simulink model "WaermepumpeGrundlageAnton"  (R2013a)
settings: Solver=ode4  StartTime=0.0  StopTime=1000  FixedStep=1e-1  RelTol=1e-3
StopFcn:
  | ClearSimple
libraries: Thermolib x98, simulink x5
(part 2 of 2)

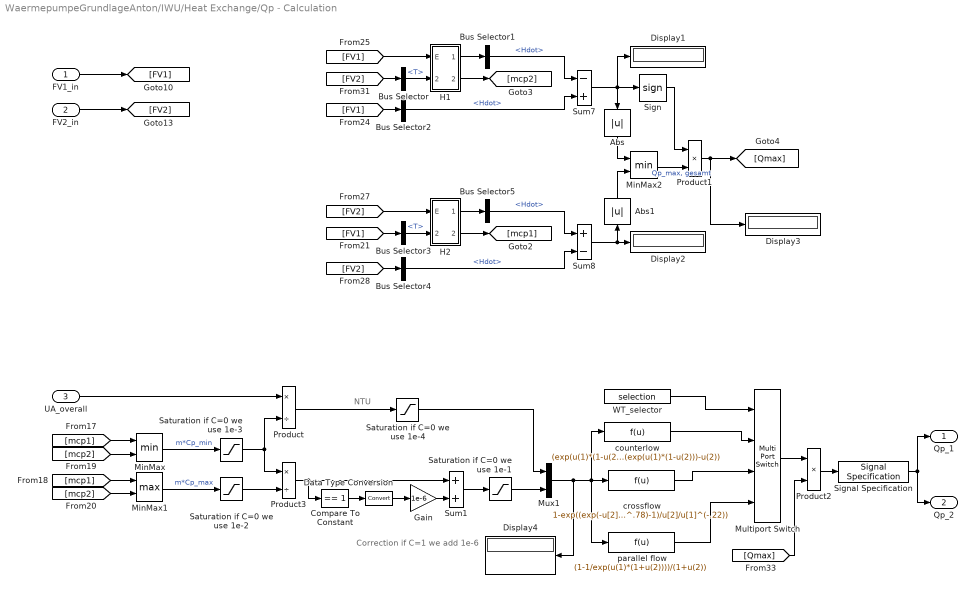
== system WaermepumpeGrundlageAnton/IWU/Heat Exchange/Qp - Calculation ==
  note: Correction if C=1
      | we add 1e-6
  note: NTU
  FV1_in : Inport
  FV2_in : Inport  Port=2
  UA_overall : Inport  Port=3
  Abs : Abs
  Abs1 : Abs
  Bus Selector : BusSelector  OutputSignals=T
  Bus Selector{1..2,4..5} (4 alike) : BusSelector  OutputSignals=Hdot
  Bus Selector3 : BusSelector  OutputSignals=T
  Compare To Constant : simulink/Logic and Bit Operations/Compare To Constant  relop===  const=1  OutDataTypeStr=uint8  ZeroCross=off
  Data Type Conversion : DataTypeConversion
  Display{1..4} (4 alike) : Display
  Gain : Gain  Gain=1e-6
  H1 : Subsystem  TreatAsAtomicUnit=on  mask(H){}
      mask Display: disp('H_g')
  H2 : Subsystem  TreatAsAtomicUnit=on  mask(H){}
      mask Display: disp('H_g')
  MinMax : MinMax  Inputs=2  SaturateOnIntegerOverflow=on  InputSameDT=on
  MinMax1 : MinMax  Function=max  Inputs=2  SaturateOnIntegerOverflow=on  InputSameDT=on
  MinMax2 : MinMax  Inputs=2  SaturateOnIntegerOverflow=on  InputSameDT=on
  Multiport Switch : MultiPortSwitch  SaturateOnIntegerOverflow=on
  Mux1 : Mux  Inputs=2
  Product : Product  Inputs=*/  SaturateOnIntegerOverflow=on  InputSameDT=on  OutDataTypeStr=Inherit: Same as first input
  Product1 : Product  SaturateOnIntegerOverflow=on  InputSameDT=on  OutDataTypeStr=Inherit: Same as first input
  Product2 : Product  SaturateOnIntegerOverflow=on  InputSameDT=on  OutDataTypeStr=Inherit: Same as first input
  Product3 : Product  Inputs=*/  SaturateOnIntegerOverflow=on  InputSameDT=on  OutDataTypeStr=Inherit: Same as first input
  Saturation if C=0 we use 1e-1 : Saturate  UpperLimit=1e19  LowerLimit=1e-19
  Saturation if C=0 we use 1e-2 : Saturate  UpperLimit=1e19  LowerLimit=1e-19
  Saturation if C=0 we use 1e-3 : Saturate  UpperLimit=1e19  LowerLimit=1e-19
  Saturation if C=0 we use 1e-4 : Saturate  UpperLimit=100  LowerLimit=1e-19
  Sign : Signum
  Signal Specification : SignalSpecification  Dimensions=1
  Sum1 : Sum  Inputs=2  SaturateOnIntegerOverflow=on  InputSameDT=on  OutDataTypeStr=Inherit: Same as first input
  Sum7 : Sum  Inputs=-+  SaturateOnIntegerOverflow=on  InputSameDT=on  OutDataTypeStr=Inherit: Same as first input
  Sum8 : Sum  Inputs=+-  SaturateOnIntegerOverflow=on  InputSameDT=on  OutDataTypeStr=Inherit: Same as first input
  WT_selector : Constant  Value=selection
  counterlow : Fcn  Expr=(exp(u(1)*(1-u(2)))-1)/(exp(u(1)*(1-u(2)))-u(2))
  crossflow : Fcn  Expr=1-exp((exp(-u[2]*u[1]^.78)-1)/u[2]/u[1]^(-.22))
  parallel flow : Fcn  Expr=(1-1/exp(u(1)*(1+u(2))))/(1+u(2))
  Qp_1 : Outport
  Qp_2 : Outport  Port=2
  wires:
  Signal Specification/1 -> Qp_2/1, Qp_1/1
  Bus Selector5/1 -> Sum8/1  "<Hdot>"
  Bus Selector4/1 -> Sum8/2  "<Hdot>"
  Bus Selector2/1 -> Sum7/2  "<Hdot>"
  Bus Selector1/1 -> Sum7/1  "<Hdot>"
  Saturation if C=0 we use 1e-1/1 -> Mux1/2
  Saturation if C=0 we use 1e-3/1 -> Product/2, Product3/1
  Saturation if C=0 we use 1e-2/1 -> Product3/2
  Sum1/1 -> Saturation if C=0 we use 1e-1/1
  Gain/1 -> Sum1/2
  Data Type Conversion/1 -> Gain/1
  Compare To Constant/1 -> Data Type Conversion/1
  Product2/1 -> Signal Specification/1
  Mux1/1 -> Display4/1, counterlow/1, parallel flow/1, crossflow/1
  Product3/1 -> Sum1/1, Compare To Constant/1
  MinMax1/1 -> Saturation if C=0 we use 1e-2/1  "m*Cp_max"
  FV1_in/1 -> [FV1]
  FV2_in/1 -> [FV2]
  Product/1 -> Saturation if C=0 we use 1e-4/1
  MinMax/1 -> Saturation if C=0 we use 1e-3/1  "m*Cp_min"
  [mcp1] -> MinMax/1
  [mcp1] -> MinMax1/1
  [mcp2] -> MinMax1/2
  [mcp2] -> MinMax/2
  [Qmax] -> Product2/2
  Multiport Switch/1 -> Product2/1
  counterlow/1 -> Multiport Switch/2
  crossflow/1 -> Multiport Switch/3
  parallel flow/1 -> Multiport Switch/4
  WT_selector/1 -> Multiport Switch/1
  Bus Selector/1 -> H1/2(Temp)  "<T>"
  Bus Selector3/1 -> H2/2(Temp)  "<T>"
  [FV2] -> Bus Selector/1
  [FV2] -> Bus Selector4/1
  [FV2] -> H2/1(E)
  [FV1] -> H1/1(E)
  [FV1] -> Bus Selector2/1
  [FV1] -> Bus Selector3/1
  Sum8/1 -> Abs1/1, Display2/1
  H2/1(FB_out) -> Bus Selector5/1
  Sum7/1 -> Abs/1, Sign/1, Display1/1
  H1/1(FB_out) -> Bus Selector1/1
  MinMax2/1 -> Product1/2  "Qp_max, gesamt"
  Sign/1 -> Product1/1
  Abs/1 -> MinMax2/1
  Abs1/1 -> MinMax2/2
  Product1/1 -> [Qmax], Display3/1
  H2/2(Cp) -> [mcp1]
  H1/2(Cp) -> [mcp2]
  Saturation if C=0 we use 1e-4/1 -> Mux1/1
  UA_overall/1 -> Product/1

== system WaermepumpeGrundlageAnton/IWU/Heat Exchange/first media ==
  Qp : Inport
  FB1_in : Inport  Port=2
  Bus Assignment : BusAssignment  AssignedSignals=Hdot
  Bus Selector : BusSelector  OutputSignals=Hdot
  H-p-State with HeatLoss : Thermolib/Thermodynamic States and Properties/H-p-State with Heat Exchange  k=k_env  A_total=A_env/4  T_env=T_env  relaxation_factor=0.01  conv_limit=TH_THERM_H_P_STATE_T_CONV_LIMIT  hm_conv_limit=TH_THERM_H_P_STATE_HM_CONV_LIMIT  n_iteration=TH_THERM_H_P_STATE_NUM_ITER_MAX  T_initial=T_initial  H_initial=0  ndot_zero_eps=TH_THERM_NDOT_MIN
  Sum7 : Sum  Inputs=2  SaturateOnIntegerOverflow=on  InputSameDT=on  OutDataTypeStr=Inherit: Same as first input
  Terminator4 : Terminator
  FB1_out : Outport
  Q_env : Outport  Port=2
  wires:
  Bus Assignment/1 -> H-p-State with HeatLoss/1
  H-p-State with HeatLoss/2 -> Q_env/1
  H-p-State with HeatLoss/1 -> FB1_out/1
  Bus Selector/1 -> Sum7/2  "<Hdot>"
  Sum7/1 -> Bus Assignment/2
  Qp/1 -> Sum7/1
  FB1_in/1 -> Bus Assignment/1, Bus Selector/1
  H-p-State with HeatLoss/3 -> Terminator4/1

== system WaermepumpeGrundlageAnton/IWU/Heat Exchange/second media ==
  Qp : Inport
  FB2_in : Inport  Port=2
  Bus Assignment : BusAssignment  AssignedSignals=Hdot
  Bus Selector : BusSelector  OutputSignals=Hdot
  H-p-State with HeatLoss1 : Thermolib/Thermodynamic States and Properties/H-p-State with Heat Exchange  k=k_env  A_total=A_env/4  T_env=T_env  relaxation_factor=0.01  conv_limit=TH_THERM_H_P_STATE_T_CONV_LIMIT  hm_conv_limit=TH_THERM_H_P_STATE_HM_CONV_LIMIT  n_iteration=TH_THERM_H_P_STATE_NUM_ITER_MAX  T_initial=T_initial  H_initial=0  ndot_zero_eps=TH_THERM_NDOT_MIN
  Sum1 : Sum  Inputs=2  SaturateOnIntegerOverflow=on  InputSameDT=on  OutDataTypeStr=Inherit: Same as first input
  Terminator4 : Terminator
  FB2_out : Outport
  Q_env : Outport  Port=2
  wires:
  Bus Selector/1 -> Sum1/2  "<Hdot>"
  Bus Assignment/1 -> H-p-State with HeatLoss1/1
  H-p-State with HeatLoss1/2 -> Q_env/1
  FB2_in/1 -> Bus Assignment/1, Bus Selector/1
  Qp/1 -> Sum1/1
  Sum1/1 -> Bus Assignment/2
  H-p-State with HeatLoss1/1 -> FB2_out/1
  H-p-State with HeatLoss1/3 -> Terminator4/1

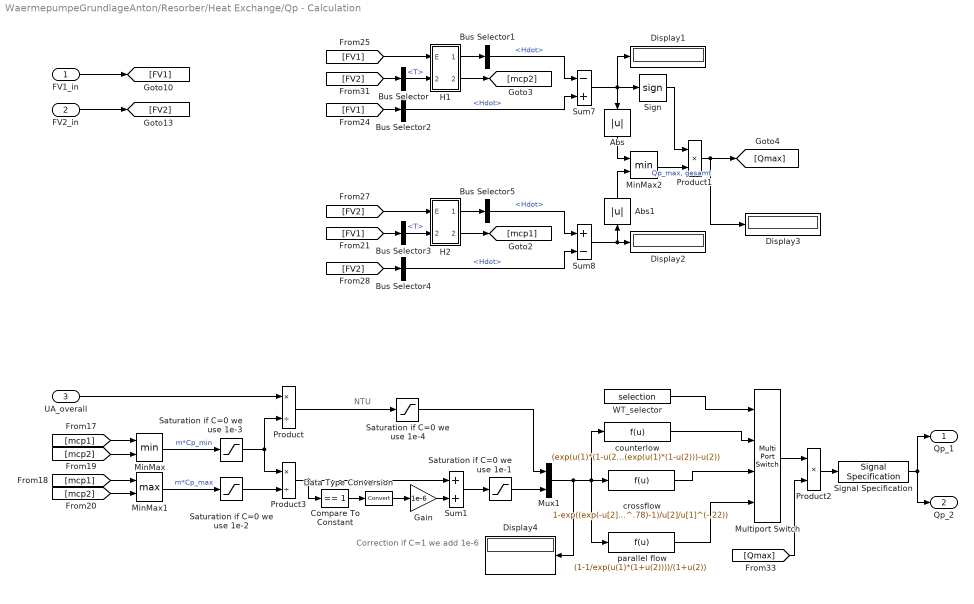
== system WaermepumpeGrundlageAnton/Resorber/Heat Exchange/Qp - Calculation ==
  note: NTU
  note: Correction if C=1
      | we add 1e-6
  FV1_in : Inport
  FV2_in : Inport  Port=2
  UA_overall : Inport  Port=3
  Abs : Abs
  Abs1 : Abs
  Bus Selector : BusSelector  OutputSignals=T
  Bus Selector{1..2,4..5} (4 alike) : BusSelector  OutputSignals=Hdot
  Bus Selector3 : BusSelector  OutputSignals=T
  Compare To Constant : simulink/Logic and Bit Operations/Compare To Constant  relop===  const=1  OutDataTypeStr=uint8  ZeroCross=off
  Data Type Conversion : DataTypeConversion
  Display{1..4} (4 alike) : Display
  Gain : Gain  Gain=1e-6
  H1 : Subsystem  TreatAsAtomicUnit=on  mask(H){}
      mask Display: disp('H_g')
  H2 : Subsystem  TreatAsAtomicUnit=on  mask(H){}
      mask Display: disp('H_g')
  MinMax : MinMax  Inputs=2  SaturateOnIntegerOverflow=on  InputSameDT=on
  MinMax1 : MinMax  Function=max  Inputs=2  SaturateOnIntegerOverflow=on  InputSameDT=on
  MinMax2 : MinMax  Inputs=2  SaturateOnIntegerOverflow=on  InputSameDT=on
  Multiport Switch : MultiPortSwitch  SaturateOnIntegerOverflow=on
  Mux1 : Mux  Inputs=2
  Product : Product  Inputs=*/  SaturateOnIntegerOverflow=on  InputSameDT=on  OutDataTypeStr=Inherit: Same as first input
  Product1 : Product  SaturateOnIntegerOverflow=on  InputSameDT=on  OutDataTypeStr=Inherit: Same as first input
  Product2 : Product  SaturateOnIntegerOverflow=on  InputSameDT=on  OutDataTypeStr=Inherit: Same as first input
  Product3 : Product  Inputs=*/  SaturateOnIntegerOverflow=on  InputSameDT=on  OutDataTypeStr=Inherit: Same as first input
  Saturation if C=0 we use 1e-1 : Saturate  UpperLimit=1e19  LowerLimit=1e-19
  Saturation if C=0 we use 1e-2 : Saturate  UpperLimit=1e19  LowerLimit=1e-19
  Saturation if C=0 we use 1e-3 : Saturate  UpperLimit=1e19  LowerLimit=1e-19
  Saturation if C=0 we use 1e-4 : Saturate  UpperLimit=100  LowerLimit=1e-19
  Sign : Signum
  Signal Specification : SignalSpecification  Dimensions=1
  Sum1 : Sum  Inputs=2  SaturateOnIntegerOverflow=on  InputSameDT=on  OutDataTypeStr=Inherit: Same as first input
  Sum7 : Sum  Inputs=-+  SaturateOnIntegerOverflow=on  InputSameDT=on  OutDataTypeStr=Inherit: Same as first input
  Sum8 : Sum  Inputs=+-  SaturateOnIntegerOverflow=on  InputSameDT=on  OutDataTypeStr=Inherit: Same as first input
  WT_selector : Constant  Value=selection
  counterlow : Fcn  Expr=(exp(u(1)*(1-u(2)))-1)/(exp(u(1)*(1-u(2)))-u(2))
  crossflow : Fcn  Expr=1-exp((exp(-u[2]*u[1]^.78)-1)/u[2]/u[1]^(-.22))
  parallel flow : Fcn  Expr=(1-1/exp(u(1)*(1+u(2))))/(1+u(2))
  Qp_1 : Outport
  Qp_2 : Outport  Port=2
  wires:
  UA_overall/1 -> Product/1
  Saturation if C=0 we use 1e-4/1 -> Mux1/1
  H1/2(Cp) -> [mcp2]
  H2/2(Cp) -> [mcp1]
  Product1/1 -> Display3/1, [Qmax]
  Abs1/1 -> MinMax2/2
  Abs/1 -> MinMax2/1
  Sign/1 -> Product1/1
  MinMax2/1 -> Product1/2  "Qp_max, gesamt"
  H1/1(FB_out) -> Bus Selector1/1
  Sum7/1 -> Display1/1, Sign/1, Abs/1
  H2/1(FB_out) -> Bus Selector5/1
  Sum8/1 -> Display2/1, Abs1/1
  [FV1] -> Bus Selector3/1
  [FV1] -> Bus Selector2/1
  [FV1] -> H1/1(E)
  [FV2] -> H2/1(E)
  [FV2] -> Bus Selector4/1
  [FV2] -> Bus Selector/1
  Bus Selector3/1 -> H2/2(Temp)  "<T>"
  Bus Selector/1 -> H1/2(Temp)  "<T>"
  WT_selector/1 -> Multiport Switch/1
  parallel flow/1 -> Multiport Switch/4
  crossflow/1 -> Multiport Switch/3
  counterlow/1 -> Multiport Switch/2
  Multiport Switch/1 -> Product2/1
  [Qmax] -> Product2/2
  [mcp2] -> MinMax/2
  [mcp2] -> MinMax1/2
  [mcp1] -> MinMax1/1
  [mcp1] -> MinMax/1
  MinMax/1 -> Saturation if C=0 we use 1e-3/1  "m*Cp_min"
  Product/1 -> Saturation if C=0 we use 1e-4/1
  FV2_in/1 -> [FV2]
  FV1_in/1 -> [FV1]
  MinMax1/1 -> Saturation if C=0 we use 1e-2/1  "m*Cp_max"
  Product3/1 -> Compare To Constant/1, Sum1/1
  Mux1/1 -> crossflow/1, parallel flow/1, counterlow/1, Display4/1
  Product2/1 -> Signal Specification/1
  Compare To Constant/1 -> Data Type Conversion/1
  Data Type Conversion/1 -> Gain/1
  Gain/1 -> Sum1/2
  Sum1/1 -> Saturation if C=0 we use 1e-1/1
  Saturation if C=0 we use 1e-2/1 -> Product3/2
  Saturation if C=0 we use 1e-3/1 -> Product3/1, Product/2
  Saturation if C=0 we use 1e-1/1 -> Mux1/2
  Bus Selector1/1 -> Sum7/1  "<Hdot>"
  Bus Selector2/1 -> Sum7/2  "<Hdot>"
  Bus Selector4/1 -> Sum8/2  "<Hdot>"
  Bus Selector5/1 -> Sum8/1  "<Hdot>"
  Signal Specification/1 -> Qp_1/1, Qp_2/1

== system WaermepumpeGrundlageAnton/Resorber/Heat Exchange/first media ==
  Qp : Inport
  FB1_in : Inport  Port=2
  Bus Assignment : BusAssignment  AssignedSignals=Hdot
  Bus Selector : BusSelector  OutputSignals=Hdot
  H-p-State with HeatLoss : Thermolib/Thermodynamic States and Properties/H-p-State with Heat Exchange  k=k_env  A_total=A_env/4  T_env=T_env  relaxation_factor=0.01  conv_limit=TH_THERM_H_P_STATE_T_CONV_LIMIT  hm_conv_limit=TH_THERM_H_P_STATE_HM_CONV_LIMIT  n_iteration=TH_THERM_H_P_STATE_NUM_ITER_MAX  T_initial=T_initial  H_initial=0  ndot_zero_eps=TH_THERM_NDOT_MIN
  Sum7 : Sum  Inputs=2  SaturateOnIntegerOverflow=on  InputSameDT=on  OutDataTypeStr=Inherit: Same as first input
  Terminator4 : Terminator
  FB1_out : Outport
  Q_env : Outport  Port=2
  wires:
  H-p-State with HeatLoss/3 -> Terminator4/1
  FB1_in/1 -> Bus Selector/1, Bus Assignment/1
  Qp/1 -> Sum7/1
  Sum7/1 -> Bus Assignment/2
  Bus Selector/1 -> Sum7/2  "<Hdot>"
  H-p-State with HeatLoss/1 -> FB1_out/1
  H-p-State with HeatLoss/2 -> Q_env/1
  Bus Assignment/1 -> H-p-State with HeatLoss/1

== system WaermepumpeGrundlageAnton/Resorber/Heat Exchange/second media ==
  Qp : Inport
  FB2_in : Inport  Port=2
  Bus Assignment : BusAssignment  AssignedSignals=Hdot
  Bus Selector : BusSelector  OutputSignals=Hdot
  H-p-State with HeatLoss1 : Thermolib/Thermodynamic States and Properties/H-p-State with Heat Exchange  k=k_env  A_total=A_env/4  T_env=T_env  relaxation_factor=0.01  conv_limit=TH_THERM_H_P_STATE_T_CONV_LIMIT  hm_conv_limit=TH_THERM_H_P_STATE_HM_CONV_LIMIT  n_iteration=TH_THERM_H_P_STATE_NUM_ITER_MAX  T_initial=T_initial  H_initial=0  ndot_zero_eps=TH_THERM_NDOT_MIN
  Sum1 : Sum  Inputs=2  SaturateOnIntegerOverflow=on  InputSameDT=on  OutDataTypeStr=Inherit: Same as first input
  Terminator4 : Terminator
  FB2_out : Outport
  Q_env : Outport  Port=2
  wires:
  H-p-State with HeatLoss1/3 -> Terminator4/1
  H-p-State with HeatLoss1/1 -> FB2_out/1
  Sum1/1 -> Bus Assignment/2
  Qp/1 -> Sum1/1
  FB2_in/1 -> Bus Selector/1, Bus Assignment/1
  H-p-State with HeatLoss1/2 -> Q_env/1
  Bus Assignment/1 -> H-p-State with HeatLoss1/1
  Bus Selector/1 -> Sum1/2  "<Hdot>"

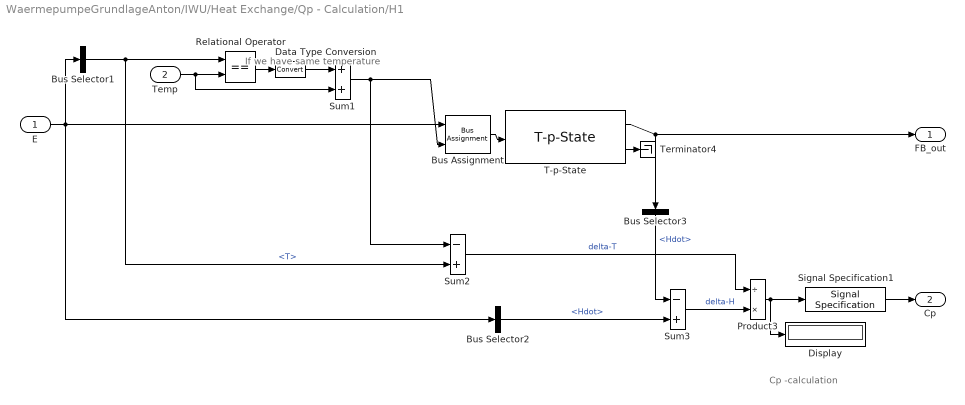
== system WaermepumpeGrundlageAnton/IWU/Heat Exchange/Qp - Calculation/H1 ==
  note: If we have same temperature
  note: Cp -calculation
  E : Inport
  Temp : Inport  Port=2
  Bus Assignment : BusAssignment  AssignedSignals=T
  Bus Selector1 : BusSelector  OutputSignals=T
  Bus Selector2 : BusSelector  OutputSignals=Hdot
  Bus Selector3 : BusSelector  OutputSignals=Hdot
  Data Type Conversion : DataTypeConversion
  Display : Display
  Product3 : Product  Inputs=/*  SaturateOnIntegerOverflow=on  InputSameDT=on  OutDataTypeStr=Inherit: Same as first input
  Relational Operator : RelationalOperator  Operator===  OutDataTypeStr=boolean
  Signal Specification1 : SignalSpecification  Dimensions=1
  Sum1 : Sum  Inputs=2  SaturateOnIntegerOverflow=on  InputSameDT=on  OutDataTypeStr=Inherit: Same as first input
  Sum2 : Sum  Inputs=-+  SaturateOnIntegerOverflow=on  InputSameDT=on  OutDataTypeStr=Inherit: Same as first input
  Sum3 : Sum  Inputs=-+  SaturateOnIntegerOverflow=on  InputSameDT=on  OutDataTypeStr=Inherit: Same as first input
  T-p-State : Thermolib/Thermodynamic States and Properties/T-p-State
  Terminator4 : Terminator
  FB_out : Outport
  Cp : Outport  Port=2
  wires:
  Signal Specification1/1 -> Cp/1
  Bus Selector3/1 -> Sum3/1  "<Hdot>"
  Bus Selector2/1 -> Sum3/2  "<Hdot>"
  Product3/1 -> Signal Specification1/1, Display/1
  Sum2/1 -> Product3/1  "delta-T"
  Sum3/1 -> Product3/2  "delta-H"
  Data Type Conversion/1 -> Sum1/1
  Relational Operator/1 -> Data Type Conversion/1
  Temp/1 -> Sum1/2, Relational Operator/2
  E/1 -> Bus Assignment/1, Bus Selector2/1, Bus Selector1/1
  T-p-State/1 -> Bus Selector3/1, FB_out/1
  Bus Assignment/1 -> T-p-State/1
  Bus Selector1/1 -> Sum2/2, Relational Operator/1  "<T>"
  Sum1/1 -> Sum2/1, Bus Assignment/2
  T-p-State/2 -> Terminator4/1

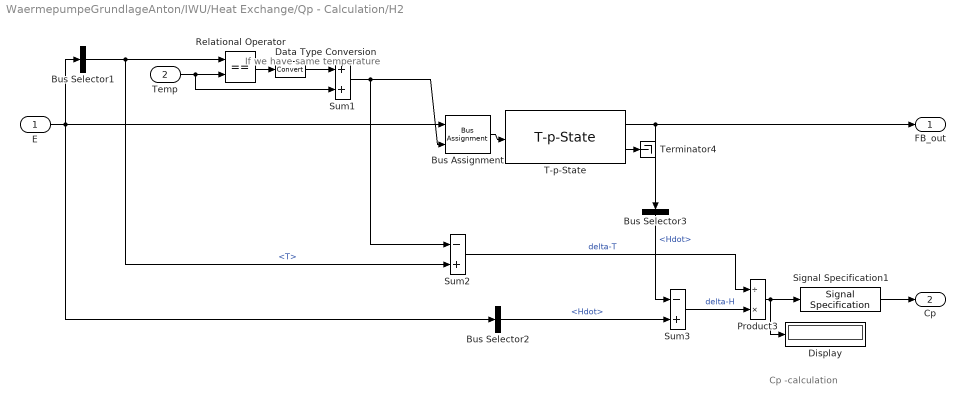
== system WaermepumpeGrundlageAnton/IWU/Heat Exchange/Qp - Calculation/H2 ==
  note: Cp -calculation
  note: If we have same temperature
  E : Inport
  Temp : Inport  Port=2
  Bus Assignment : BusAssignment  AssignedSignals=T
  Bus Selector1 : BusSelector  OutputSignals=T
  Bus Selector2 : BusSelector  OutputSignals=Hdot
  Bus Selector3 : BusSelector  OutputSignals=Hdot
  Data Type Conversion : DataTypeConversion
  Display : Display
  Product3 : Product  Inputs=/*  SaturateOnIntegerOverflow=on  InputSameDT=on  OutDataTypeStr=Inherit: Same as first input
  Relational Operator : RelationalOperator  Operator===  OutDataTypeStr=boolean
  Signal Specification1 : SignalSpecification  Dimensions=1
  Sum1 : Sum  Inputs=2  SaturateOnIntegerOverflow=on  InputSameDT=on  OutDataTypeStr=Inherit: Same as first input
  Sum2 : Sum  Inputs=-+  SaturateOnIntegerOverflow=on  InputSameDT=on  OutDataTypeStr=Inherit: Same as first input
  Sum3 : Sum  Inputs=-+  SaturateOnIntegerOverflow=on  InputSameDT=on  OutDataTypeStr=Inherit: Same as first input
  T-p-State : Thermolib/Thermodynamic States and Properties/T-p-State
  Terminator4 : Terminator
  FB_out : Outport
  Cp : Outport  Port=2
  wires:
  Signal Specification1/1 -> Cp/1
  Sum1/1 -> Bus Assignment/2, Sum2/1
  Bus Selector1/1 -> Relational Operator/1, Sum2/2  "<T>"
  Bus Assignment/1 -> T-p-State/1
  T-p-State/1 -> FB_out/1, Bus Selector3/1
  E/1 -> Bus Selector1/1, Bus Selector2/1, Bus Assignment/1
  Temp/1 -> Relational Operator/2, Sum1/2
  Relational Operator/1 -> Data Type Conversion/1
  Data Type Conversion/1 -> Sum1/1
  Sum3/1 -> Product3/2  "delta-H"
  Sum2/1 -> Product3/1  "delta-T"
  Product3/1 -> Signal Specification1/1, Display/1
  Bus Selector2/1 -> Sum3/2  "<Hdot>"
  Bus Selector3/1 -> Sum3/1  "<Hdot>"
  T-p-State/2 -> Terminator4/1

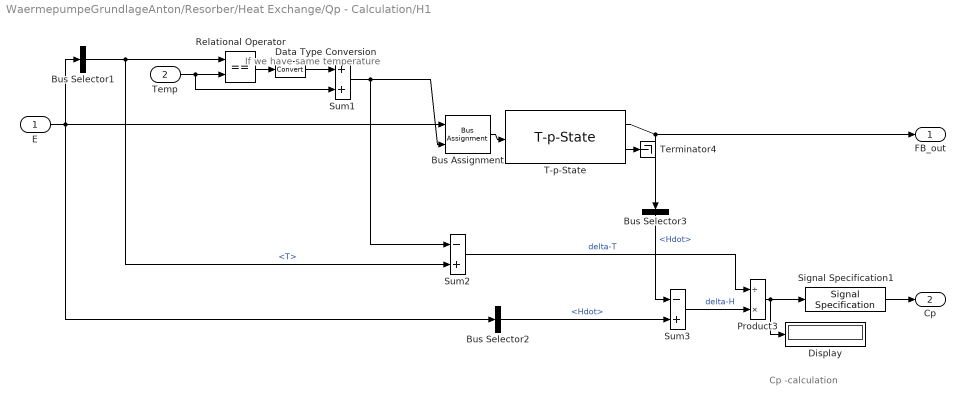
== system WaermepumpeGrundlageAnton/Resorber/Heat Exchange/Qp - Calculation/H1 ==
  note: Cp -calculation
  note: If we have same temperature
  E : Inport
  Temp : Inport  Port=2
  Bus Assignment : BusAssignment  AssignedSignals=T
  Bus Selector1 : BusSelector  OutputSignals=T
  Bus Selector2 : BusSelector  OutputSignals=Hdot
  Bus Selector3 : BusSelector  OutputSignals=Hdot
  Data Type Conversion : DataTypeConversion
  Display : Display
  Product3 : Product  Inputs=/*  SaturateOnIntegerOverflow=on  InputSameDT=on  OutDataTypeStr=Inherit: Same as first input
  Relational Operator : RelationalOperator  Operator===  OutDataTypeStr=boolean
  Signal Specification1 : SignalSpecification  Dimensions=1
  Sum1 : Sum  Inputs=2  SaturateOnIntegerOverflow=on  InputSameDT=on  OutDataTypeStr=Inherit: Same as first input
  Sum2 : Sum  Inputs=-+  SaturateOnIntegerOverflow=on  InputSameDT=on  OutDataTypeStr=Inherit: Same as first input
  Sum3 : Sum  Inputs=-+  SaturateOnIntegerOverflow=on  InputSameDT=on  OutDataTypeStr=Inherit: Same as first input
  T-p-State : Thermolib/Thermodynamic States and Properties/T-p-State
  Terminator4 : Terminator
  FB_out : Outport
  Cp : Outport  Port=2
  wires:
  T-p-State/2 -> Terminator4/1
  Sum1/1 -> Bus Assignment/2, Sum2/1
  Bus Selector1/1 -> Relational Operator/1, Sum2/2  "<T>"
  Bus Assignment/1 -> T-p-State/1
  T-p-State/1 -> FB_out/1, Bus Selector3/1
  E/1 -> Bus Selector1/1, Bus Selector2/1, Bus Assignment/1
  Temp/1 -> Relational Operator/2, Sum1/2
  Relational Operator/1 -> Data Type Conversion/1
  Data Type Conversion/1 -> Sum1/1
  Sum3/1 -> Product3/2  "delta-H"
  Sum2/1 -> Product3/1  "delta-T"
  Product3/1 -> Display/1, Signal Specification1/1
  Bus Selector2/1 -> Sum3/2  "<Hdot>"
  Bus Selector3/1 -> Sum3/1  "<Hdot>"
  Signal Specification1/1 -> Cp/1

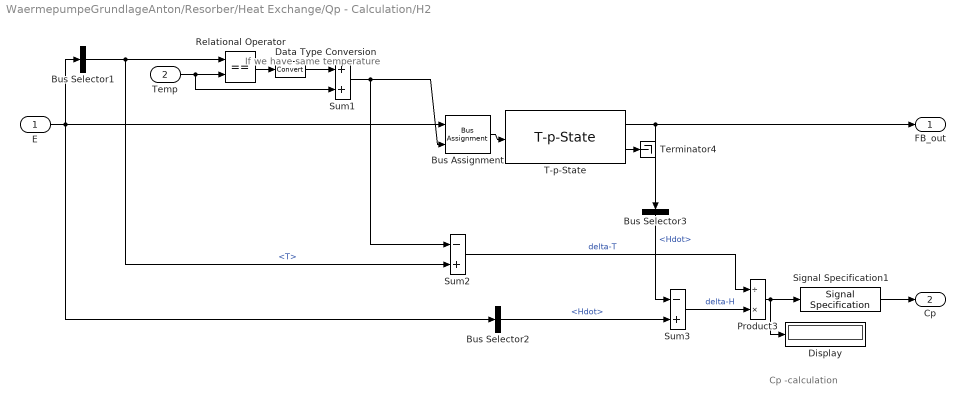
== system WaermepumpeGrundlageAnton/Resorber/Heat Exchange/Qp - Calculation/H2 ==
  note: If we have same temperature
  note: Cp -calculation
  E : Inport
  Temp : Inport  Port=2
  Bus Assignment : BusAssignment  AssignedSignals=T
  Bus Selector1 : BusSelector  OutputSignals=T
  Bus Selector2 : BusSelector  OutputSignals=Hdot
  Bus Selector3 : BusSelector  OutputSignals=Hdot
  Data Type Conversion : DataTypeConversion
  Display : Display
  Product3 : Product  Inputs=/*  SaturateOnIntegerOverflow=on  InputSameDT=on  OutDataTypeStr=Inherit: Same as first input
  Relational Operator : RelationalOperator  Operator===  OutDataTypeStr=boolean
  Signal Specification1 : SignalSpecification  Dimensions=1
  Sum1 : Sum  Inputs=2  SaturateOnIntegerOverflow=on  InputSameDT=on  OutDataTypeStr=Inherit: Same as first input
  Sum2 : Sum  Inputs=-+  SaturateOnIntegerOverflow=on  InputSameDT=on  OutDataTypeStr=Inherit: Same as first input
  Sum3 : Sum  Inputs=-+  SaturateOnIntegerOverflow=on  InputSameDT=on  OutDataTypeStr=Inherit: Same as first input
  T-p-State : Thermolib/Thermodynamic States and Properties/T-p-State
  Terminator4 : Terminator
  FB_out : Outport
  Cp : Outport  Port=2
  wires:
  T-p-State/2 -> Terminator4/1
  Bus Selector3/1 -> Sum3/1  "<Hdot>"
  Bus Selector2/1 -> Sum3/2  "<Hdot>"
  Product3/1 -> Display/1, Signal Specification1/1
  Sum2/1 -> Product3/1  "delta-T"
  Sum3/1 -> Product3/2  "delta-H"
  Data Type Conversion/1 -> Sum1/1
  Relational Operator/1 -> Data Type Conversion/1
  Temp/1 -> Sum1/2, Relational Operator/2
  E/1 -> Bus Assignment/1, Bus Selector2/1, Bus Selector1/1
  T-p-State/1 -> Bus Selector3/1, FB_out/1
  Bus Assignment/1 -> T-p-State/1
  Bus Selector1/1 -> Sum2/2, Relational Operator/1  "<T>"
  Sum1/1 -> Sum2/1, Bus Assignment/2
  Signal Specification1/1 -> Cp/1
